simulink model "BaseEngineController_LS_128"  (Simulink 7.7)
settings: Solver=FixedStepDiscrete  StartTime=0.0  StopTime=10.0  RelTol=1e-3
PreLoadFcn:
  | try, eval([bdroot '_setup']); catch, eval('model_setup', ''); end
InitFcn:
  | try, eval([bdroot '_setup']); catch, eval('model_setup', ''); end
undefined symbols (not defined in the file): ECU565, High, motohawk_build_version, motohawk_trunc_name, motohawk_vardec_config_group, motohawk_vardec_path, True
libraries: MotoHawk_lib x1418, motohawk_control_primitives_lib x183, motohawk_engine_lib x32, simulink x21, motohawk_annotations_lib x9, AutoDoc_lib x8, simulink_extras x4, motohawk_ccp_examples_lib x1, motohawk_control_primitives_motoshare_lib x1
(part 1 of 27)
Description:
  | MI07 SECM48
CloseFcn:
  | rtwprivate ssgencode ModelCloseRequest BaseEngineController_A02
settings Model: MotoHawkBuildVersion=035  MotoHawkBuildStats=struct('TotalFLASH',{373552},'TotalEEPROM',{1254},'TotalRAM',{26040},'AppFLASH',{154160},'AppEEPROM',{1080},'AppRAM',{7766},'HeapRAM',{4096},'BuildSuccessCount',{48},'BuildErrorCount',{105},'OSRAM',{4962},'StackRAM',{9216},'FgndTimeStackSize',{4096},'FgndAngleStackSize',{1024},'BgndStackSize',{2048},'IdleStackSize',{1024},'InterruptStackSize',{1024},'RTWBlockIOSize',{2192},'RTWDWorkSize',{1776},'RTWPrevZCSize',{0},'VolatileSize',{1668},'NonVolatileSize',{1080},'ConstantSize',{18616},'NonVolatileFormatID',{32179})  MotoHawkModelSavedName=BaseEngineController_LS_128  MotoHawkModelGUID=a749ec14-8a37-4ecf-bb-ef-07-f5-29-2a-95  MotoHawkModelOpenTime=2022 11 22 13 19 39.99  MotoHawkModelElapsedTime=-3851959716.408  MotoHawkBuildGUID=70e4bce9-a719-451e-bc-76-a9-56-b2-7d-46  MotoHawkBuildInfo=struct('model_name',{'BaseEngineController_LS_128'},'motohawk_version',{'2011a_sp0.184'},'motohawk_component_version',{'0.0.7'},'matlab_version',{'7.12.0'},'build_version',{'034'},'module_type',{'ECU565-128'},'layout_type',{'DEV'},'processor_family',{'PPC'},'processor_type',{'MPC565'},'toolchain_vendor',{'gcc-powerpc-eabi'},'toolchain_version',{'4.4.0'},'component',{0},'archive_file',{'PCM128.a'},'enable_build',{1},'fptype',{0},'flash_size',{1048576},'ee_size',{8192},'ram_size',{36864},'decram_size',{4096},'module_memory_def',{'MPC565_ModMemoryDef_Dev'},'eri_table0_rev',{9},'max_eri_table_size',{65535},'use_debug_vardecs',{1},'use_info_vardecs',{1},'fgnd_base_period_ms',{5},'bgnd_base_period_ms',{50},'root_build_dir',{'C:\Users\maxar\Documents\GitHub\Engine-Controller\EngineController_128Branch'},'build_dir',{'C:\Users\maxar\Documents\GitHub\Engine-Controller\EngineController_128Branch\BaseEngineController_LS_128_Build'},'dll_name',{'BaseEngin_034'},'srz_name',{'BaseEngineController_LS_128_034'},'fgnd_stack_size',{4096},'fgnd_angle_stack_size',{0},'bgnd_stack_size',{1024},'idle_stack_size',{1024},'irq_stack_size',{1280},'heap_size',{2048},'heap_margin',{409},'install_dll_dir',{'c:\ecufiles\tdbdll'},'install_srz_dir',{'C:\ECUFiles\Programs\'},'app_int_stack_size',{1024},'shutdown_stack_size',{1024},'mingw_dir',{'C:\PROGRA~2\Woodward\DEVELO~1\TOOLCH~1\GCC\win32-pe\4_4_0\'},'motohawk_dir',{'C:\PROGRA~2\Woodward\MCS\MotoHawk\2011A_~1.184'},'toolchain_dir',{'C:\Program Files (x86)\Woodward\DevelopmentTools\Toolchains\GCC\powerpc-eabi\4_4_0\'},'matlab_root',{'E:\MATLAB\2011a'},'model_guid',{'a749ec14-8a37-4ecf-bb-ef-07-f5-29-2a-95'},'build_guid',{'70e4bce9-a719-451e-bc-76-a9-56-b2-7d-46'},'token_guid',{'DD8AD11F95A6FC42BFF9AC780840E4B4'})  RegisteredStructs=struct('Name',{'FreezeFrame','FreezeFrames'},'Data',{struct('Name',{int32(0)},'Code',{int32(0)},'Var1',{int32(0)},'Var2',{int32(0)},'Var3',{int32(0)},'Var4',{int32(0)},'Var5',{int32(0)},'Var6',{int32(0)},'Var7',{int32(0)},'Var8',{int32(0)},'Var9',{int32(0)},'Var10',{int32(0)}),struct('Name',{int32(0)},'Code',{int32(0)},'Var1',{int32(0)},'Var2',{int32(0)},'Var3',{int32(0)},'Var4',{int32(0)},'Var5',{int32(0)},'Var6',{int32(0)},'Var7',{int32(0)},'Var8',{int32(0)},'Var9',{int32(0)},'Var10',{int32(0)})},'Enums',{{{'None','APP_Sensors_Conflict','CamEdgesFault','CamSyncFault','CrankEdgesFault','CrankSyncFault','ECTOverTempFault','ECTRangeHigh','ECTRangeLow','ECT_IR_Fault','EST1_Open','EST1_Short','EST2_Open','EST2_Short','EST3_Open','EST3_Short','EST4_Open','EST4_Short','EST5_Open','EST5_Short','EST6_Open','EST6_Short','EST7_Open','EST7_Short','EST8_Open','EST8_Short','ETCSpringTest','ETC_Open_Fault','ETC_Sticking','FuelAdaptRangeHi','FuelAdaptRangeLow','FuelTempRangeHigh','FuelTempRangeLow','HBridgeFault_ETC','HardOverspeed','IATRangeHigh','IATRangeLow','IAT_IR_Fault','Inj1Open','Inj2Open','Inj3Open','Inj4Open','Inj5Open','Inj6Open','Inj7Open','Inj8Open','LSDFault_FuelPump','LSDFault_MIL','LSOFault_VVT','MAFRangeHigh','MAFRangeLow','MAPRangeHigh','MAPRangeLow','MAPTimeRangeHigh','MAPTimeRangeLow','MAP_IR_HI','MAP_IR_LO','MAP_STICKING','MediumOverspeed','O2FailedLean','O2FailedRich','O2NotActive','OilTempRangeHigh','OilTempRangeLow','SensVoltRangeHigh','SensVoltRangeLow','SoftOverspeed','SysVoltRangeHigh','SysVoltRangeLow','TPS_Sensors_Conflict'}},{{'None','CamEdgesFault','CamSyncFault','CrankEdgesFault','CrankSyncFault','ECTOverTempFault','ECTRangeHigh','ECTRangeLow','ECTSevereOverTempFault','EGRSenseRangeHigh','EGRSenseRangeLow','EST1_Open','EST1_Short','EST2_Open','EST2_Short','ETCSpringTest','ETC_Open_Fault','ETC_Sticking','FuelAdaptRangeHi','FuelAdaptRangeLow','FuelPresHigh_Fault','FuelPresLow_Fault','FuelPresRangeHigh','FuelPresRangeLow','FuelSensRangeHigh','FuelSensRangeLow','HBridgeFault_ETC','HardOverspeed','IATRangeHigh','IATRangeLow','Inj1Open','Inj2Open','LSDFault_FuelPump','LSDFault_OilPump','LSDFault_OxygenHeater','MAFRangeHigh','MAFRangeLow','MAPRangeHigh','MAPRangeLow','MAPTimeRangeHigh','MAPTimeRangeLow','MAP_IR_HI','MAP_IR_LO','MAP_STICKING','MediumOverspeed','NoOil_Fault','O2FailedLean','O2FailedRich','O2NotActive','O2_PostCatRangeHigh','O2_PostCatRangeLow','OilPresRangeHigh','OilPresRangeLow','SensVoltRangeHigh','SensVoltRangeLow','SoftOverspeed','SysVoltLow_Fault','SysVoltRangeHigh','SysVoltRangeLow','TPS1AdaptHiMax','TPS1AdaptHiMin','TPS1AdaptLoMax','TPS1AdaptLoMin','TPS1RangeHigh','TPS1RangeLow','TPS2AdaptHiMax','TPS2AdaptHiMin','TPS2AdaptLoMax','TPS2AdaptLoMin','TPS2RangeHigh','TPS2RangeLow','TPS_Sensors_Conflict'}}})  Creator=dbocci  LastModifiedBy=maxar
settings OptimizationCC: InlineParams=on  InitFltsAndDblsToZero=on  OptimizeModelRefInitCode=on  LifeSpan=1
settings DebuggingCC: SolverPrmCheckMsg=none  InheritedTsInSrcMsg=none  TasksWithSamePriorityMsg=none  StrictBusMsg=Warning
settings HardwareCC: ProdEndianess=BigEndian  ProdHWDeviceType=Specified
settings RTWCC: SystemTargetFile=motohawk_ert_rtw.tlc  TLCOptions="-aCustomNonFinites=\"motohawk_genrtnonfinite.tlc\""  MakeCommand=motohawk_make_rtw  TemplateMakefile=motohawk_ert_rtw.tmf  Description=MotoHawk(tm) Rapid Prototyping  ProcessScript=motohawk_ert_rtw_make_rtw_hook
settings CodeAppCC: IgnoreCustomStorageClasses=off  MaxIdLength=100  CustomSymbolStrField=$H$N$M
settings STFCustomTargetCC: FunctionExecutionProfile=off  ModelReferenceCompliant=off  CombineOutputUpdateFcns=on  ERTCustomFileBanners=on  SupportContinuousTime=off  SupportNonInlinedSFcns=off  SystemTargetFile=motohawk_ert_rtw.tlc
settings ERTTargetCC: FunctionExecutionProfile=off  MultiwordLength=2048  ModelReferenceCompliant=off  ParMdlRefBuildCompliant=off  CompOptLevelCompliant=off  ERTFirstTimeCompliant=off  ModelStepFunctionPrototypeControlCompliant=off  CPPClassGenCompliant=off  ERTCustomFileTemplate=example_file_process.tlc  ConvertIfToSwitch=off

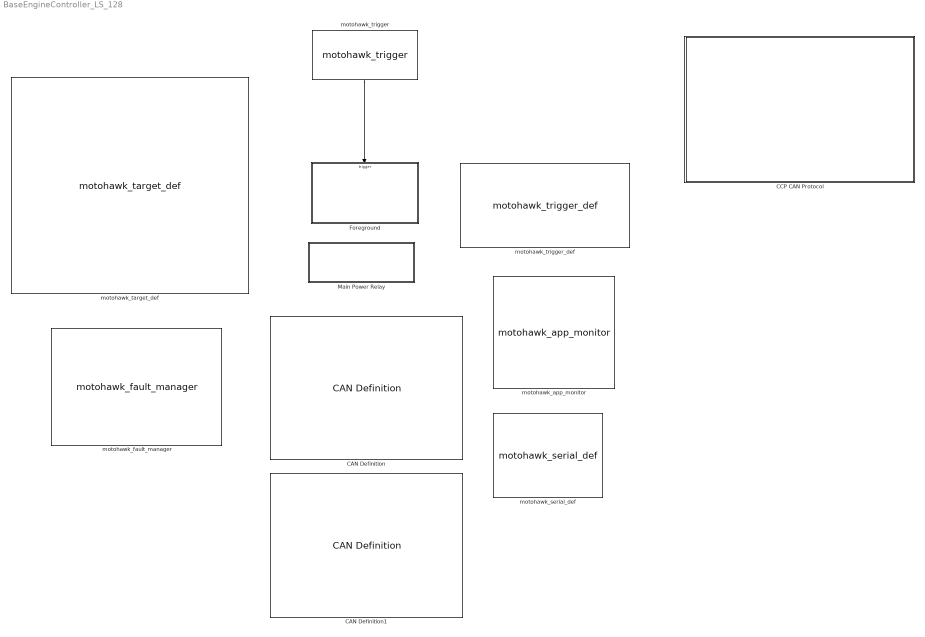
== system BaseEngineController_LS_128 ==
  CAN Definition : MotoHawk_lib/CAN Blocks/CAN Definition  Priority=-100  nam=['CAN_1']  text_resource=CAN1  code_resource=NONE  val_resource=-1  target=ECU565-128  bus=-2  btime=500 kbaud  pre=1  prop=0  pseg1=0  pseg2=0  resyn=0  tx_queue_size=16  rx_queue_size=16  use_protocol=on  city_id=hex2dec('B')  access_level=4  mototune_group='System | System Config | Communication Config'
  CAN Definition1 : MotoHawk_lib/CAN Blocks/CAN Definition  Priority=-100  nam=['CAN_2']  text_resource=CAN2  code_resource=NONE  val_resource=-1  target=ECU565-128  bus=-2  btime=500 kbaud  pre=1  prop=0  pseg1=0  pseg2=0  resyn=0  tx_queue_size=16  rx_queue_size=16  use_protocol=on  city_id=hex2dec('B')  access_level=4  mototune_group='System | System Config | Communication Config'
  CCP CAN Protocol : Subsystem  AncestorBlock=MotoHawk_lib/CCP Slave/CCP CAN Protocol  mask(MotoHawk CCP CAN Protocol Handler){image_file='ccp.jpg', mtninstance='CCP1', stataddr=hex2dec('31'), channel_name='CAN_1', channel=-2, rxid=hex2dec('18ef0231'), rxidtype=1, rxidmasknom=hex2dec('1fffffff'), txid=hex2dec('18ef3102'), txidtype=1, daqs=10, odts=8, nvodt=2, send_cpb_resp=on, use_mototune_group=on, mototune_group=['System | CCP | ', motohawk_get_param_ws(gcb, 'mtninstance')]}
      mask prompts: image_file "imfileImage File"; mtninstance "CCP Handler Instance Name (unique string)"; stataddr "CCP Station Address (16 bit integer)"; channel_name "CAN Channel Name"; channel "CAN Channel (integer)"; rxid "Receive ID (CRO)"; rxidtype "Receive ID Type (0=Std, 1=Ext)"; rxidmasknom "Receive ID Mask"; txid "Transmit ID (DTO/DAQ)"; txidtype "Transmit ID Type (0=Std, 1=Ext)"; daqs "Total Number of DAQs [1-253]"; odts "Total Number of Object Descriptors (ODT ) per DAQ [1-253]"; nvodt "Store ODTs in Non Volatile (0=RAM, 1=EEPROM, 2=CAL)"; send_cpb_resp "Send "Command Processor Busy" response prior to long memory writes"; use_mototune_group "------ Show MotoTune Group ------"; mototune_group "MotoTune Group String"
      mask help:
      | Handle a CCP connection via CAN.
      |
      | The list of DAQ Triggers is pre-selected to:
      |  o FGND_RTI_PERIODIC
      |  o FGND_2XRTI_PERIODIC
      |  o FGND_10XRTI_PERIODIC
      |  o FGND_20XRTI_PERIODIC
      |  o BGND_BASE_PERIODIC
      |  o BGND_BASEx2_PERIODIC
      |  o BGND_BASEx10_PERIODIC
      |  o ONE_SECOND_EVENT
      |
      | The CCP Command packets are responded to in the CAN interrupt in which they occur.
      | If you would like other triggering behavior, please utilize the CCP CAN Protocol External Trig
      | block from the CCP Slave Library.
      |
      | Support operations:
      | Upload Calibrations
      | Download Calibrations
      | Data Acquisition
      | Seed and Key security
      |
      | Not Supported:
      | Flashing operations
      |
      | --------------------------------------------------------------------------------
      | Copyright 2010 Woodward.  All Rights Reserved.
      mask init:
      | block = gcb;
      | try,
      | 	img = imread(image_file);
      | 	%motohawk_block_image(gcb, image_file);
      | catch,
      | 	img = imread('image_not_found.jpg');
      | end
      | 
      | if channel > -1
      | 	%% Automatically upgrade the nam parameter if the bus is currently set to a channel number
      | 	bus_expr = get_param(block, 'channel');
      | 	% Note, the set_param within the upgrade function will fail, we do the set_param next
      | 	[nam,expr] = motohawk_upgrade_can_name('', channel, bus_expr);
      | 
      | 	try
      | 		set_param(block, 'channel_name', expr, 'channel', '-2');
      | 	end
      | end
      | 
      | e = {'(std)','(ext)'};
      | o = {'RAM','EEPROM','CAL'};
      | 
      | if((nvodt > 2) || (nvodt < 0))
      | 	set_param(gcb,'nvodt','0');	
      | end
      | 
      | nvlbl = ['ODT Storage: ' o{nvodt+1}];
      | 
      | reqbits = hex2dec('1fffffff'); 
      | rxidmask = bitand(uint32(rxidmasknom),uint32(reqbits));
      | rxlbl = sprintf('\\fontname{courier new}Chan  : %s\\newlineRx ID : 0x%08x %s\\newlineID Adj: 0x%08x', motohawk_tex(channel_name),rxid,e{rxidtype+1}, double(bitxor(uint32(rxidmask),uint32(reqbits))));
      | txlbl = sprintf('\\fontname{courier new}Chan  : %s\\newlineTx ID : 0x%08x %s\\newline ', motohawk_tex(channel_name),txid,e{txidtype+1});
      settings: MoveFcn=%motohawk_block_image(gcb, motohawk_get_param_ws(gcb, 'image_file'));
      mask Help: eval('motohawk_block_help(get_param(gcb,''MaskType''))');
      mask CallbackString: |||||||||||||motohawk_set_param([gcb '/CCP CAN Protocol External Trig1'], 'send_cpb_resp', get_param(gcb, 'send_cpb_resp'));|motohawk_calibration_visible(gcb, 'use_mototune_group');|
      mask Display:
      | patch([0 0 1 1], [0 1 1 0], [220/255 220/255 220/255]);
      | patch([0 0 1 1], [0 0.075 0.075 0], [230/255 0/255 0/255]);
      | patch([0 0 1 1], [0.025 0.05 0.05 0.025], [150/255 0/255 0/255]);
      | patch([0 0 1 1], [0 0.025 0.025 0], [0/255 0/255 0/255]);
      | image(img,[0.05 0.3 0.55 0.7]);
      | 
      | text(0.99,0.57,['\fontname{Arial}\fontsize{18}\bfCCP Handler\fontsize{12}\newline\rmInstance: ' strrep(mtninstance,'_','\_') '\newlineStation Addr: ' sprintf('0x%04x',stataddr) '\newlineDAQs: ' sprintf('%g',daqs) '\newlineODTs: ' sprintf('%g',odts) '\newline' nvlbl],'texmode','on','HorizontalAlignment','Right');
      | 
      | text(0.01,0.22,['\fontname{Arial}\fontsize{18}\bfRx\fontsize{12}\newline\rm' rxlbl],'texmode','on','HorizontalAlignment','Left');
      | text(0.99,0.22,['\fontname{Arial}\fontsize{18}\bfTx\fontsize{12}\newline\rm' txlbl],'texmode','on','HorizontalAlignment','Right');
  Foreground : Subsystem  TreatAsAtomicUnit=on
      settings: RTWSystemCode=Function  RTWFcnNameOpts=Use subsystem name  RTWFileNameOpts=Use subsystem name
  Main Power Relay : Subsystem  AncestorBlock=MotoHawk_lib/Extra Development Blocks/Main Power Relay  mask(MotoHawk Main Power Relay Control){on_delay_count=2, off_delay_count=5, group='System | Main Power Relay'}
      mask prompts: on_delay_count "On Delay Count"; off_delay_count "Off Delay Count"; group "MotoTune Group"
      mask help:
      | This block provides basic control of the main power relay, by following the ECUP voltage input pin.
      |
      | Regardless of where the block is placed in a design, the strategy will execute every 50ms with background priority.
      |
      | Note that this block is simply composed of other primitive MotoHawk blocks and may be used as a starting point for a more complicated strategy.
      |
      | On Delay:  Once the ECU power goes high, after this period, the Main Power Relay will be turned on.
      | Off Delay:  Once the ECU power goes low, after this period, the Main Power Relay will be turned off.
      |
      | Note that one tick before MPRD is turned off, non-volatile variables will be stored, and the Shutdown event will be posted.  It is not necessary to use the Shutdown event.
      |
      | To delay shutdown based on Foreground events, use a data storage write block 'ShutDownTasksComplete' set as a boolean in the Foreground controller to initiate actual shutdown following completion of the tasks.
      |
      | ---------------------------------------------------------------------
      | Copyright 2005 MotoTron, Inc.  All Rights Reserved.
      mask init:
      | on_delay_lbl = sprintf('\nOn Delay: %d ms', on_delay_count * 50);
      | off_delay_lbl = sprintf('\nOff Delay: %d ms', off_delay_count * 50);
      mask Help: eval('motohawk_block_help(get_param(gcb,''MaskType''))');
      mask Display:
      | patch([0 0 1 1], [0 1 1 0], [220/255 220/255 220/255])
      | patch([0 0 1 1], [0 0.075 0.075 0], [230/255 0/255 0/255])
      | patch([0 0 1 1], [0.025 0.05 0.05 0.025], [150/255 0/255 0/255])
      | patch([0 0 1 1], [0 0.025 0.025 0], [0/255 0/255 0/255])
      | 
      | disp(['Main Power Relay' on_delay_lbl off_delay_lbl]);
  motohawk_app_monitor : MotoHawk_lib/System Debug Blocks/motohawk_app_monitor  fgnd_stack_margin=512  fgnd_angle_stack_margin=256  bgnd_stack_margin=256  idle_stack_margin=256  irq_stack_margin=128  heap_margin=256  cpu_margin=10  init_enable=Enabled  pause_point=Do Not Pause on Startup
  motohawk_fault_manager : MotoHawk_lib/Fault Management Blocks/motohawk_fault_manager  storage=FLASH  read_level=1  write_level=1  clear_level=1  xytype=uint16  mototune_group=motohawk_vardec_path(gcb)
  motohawk_serial_def : MotoHawk_lib/Serial I//O Blocks/motohawk_serial_def  res_name=[]  text_resource=RS485  code_resource=NONE  val_resource=-1  target=ECU565-128  resource_enum_str=(None)=-1,RS485=113  use_mototune=on  baud=9600  tx_queue_size=16  rx_queue_size=16
  motohawk_target_def : MotoHawk_lib/motohawk_target_def  Priority=-65535  target=ECU565-128  layout=DEV  fptype=single (32 bits)  fgnd_stack_size=4*1024  fgnd_angle_stack_size=0  bgnd_stack_size=1*1024  idle_stack_size=1024  irq_stack_size=1280  app_int_stack_size=1024  shutdown_stack_size=1024  heap_size=2*1024  show_margins=off  fgnd_stack_margin=(3*1024) * 0.1  fgnd_angle_stack_margin=0  bgnd_stack_margin=(2*1024) * 0.1  idle_stack_margin=(1024) * 0.1  irq_stack_margin=(1536) * 0.1  app_int_stack_margin=(1024) * 0.1  shutdown_stack_margin=(1024) * 0.1  heap_margin=(4*1024) * 0.1  comp_name=bdroot  comp_img='mh.jpg'  comp_security=No Encryption  comp_build_pass='mhbuild'  comp_sim_pass='mhsim'  comp_multi=off  show_filenames=on  dll_name=motohawk_trunc_name(bdroot, ['_' motohawk_build_version], 13)  srz_name=motohawk_trunc_name(bdroot, ['_' motohawk_build_version], 50)  build_dir=''  comp_dir='.'
  motohawk_trigger : MotoHawk_lib/Trigger Blocks/motohawk_trigger  Tag=Trigger  Priority=0  trigger=FGND_RTI_PERIODIC  function_name=Trigger_FGND_RTI_PERIODIC_11578p0004  priority_order=0  inherited=off  run_disabled=off  override_app_monitor=off  target=ECU565_128
  motohawk_trigger_def : MotoHawk_lib/Trigger Blocks/motohawk_trigger_def  fgnd_rti_rate=5000  bgnd_base_multiple=10  read_level=1  write_level=1  mototune_group='System | System Config | Trigger Config'
  wires:
  motohawk_trigger/1 -> Foreground/Trigger

== system BaseEngineController_LS_128/CCP CAN Protocol ==
  CCP CAN Protocol External Trig1 : MotoHawk_lib/CCP Slave/CCP CAN Protocol External Trig  SystemSampleTime=-1  image_file=image_file  mtninstance=mtninstance  stataddr=stataddr  channel_name=channel_name  channel=channel  rxid=rxid  rxidtype=rxidtype  rxidmasknom=rxidmasknom  txid=txid  txidtype=txidtype  daqs=daqs  odts=odts  nvodt=nvodt  send_cpb_resp=on  use_mototune_group=off  mototune_group=mototune_group
  CCP Triggers : motohawk_ccp_examples_lib/CCP Triggers  SystemSampleTime=-1
      link override motohawk_trigger: trigger=FGND_5XRTI_PERIODIC  function_name=Trigger_FGND_5XRTI_PERIODIC_23675p0006  target=ECU555_80
      link override motohawk_trigger2: trigger=FGND_MID_TDC_EVENT  function_name=Trigger_FGND_MID_TDC_EVENT_23677p0006  target=ECU555_80
  motohawk_trigger1 : MotoHawk_lib/Trigger Blocks/motohawk_trigger  Tag=Trigger  trigger=IDLE_EVENT  function_name=Trigger_IDLE_EVENT_9p001  priority_order=255  inherited=on  run_disabled=off  override_app_monitor=on  target=ECU565_128
  wires:
  motohawk_trigger1/1 -> CCP CAN Protocol External Trig1/1
  CCP Triggers/1 -> CCP CAN Protocol External Trig1/2

== system BaseEngineController_LS_128/Foreground ==
  f : TriggerPort  TriggerType=function-call
  Control : Subsystem  mask(Display Image File){image_file='pcm555.jpg'}
      mask prompts: image_file "Image File"
      mask help:
      | Enter an image file on the current MATLAB path to display on this block.
      |
      | Double-clicking this block opens the contents of the subsystem.  Right-click and select 'Mask parameters...' to select a new image file.
      |
      | To use just the mask of this block in a model, but supply your own contents, break the link to the library.
      mask init:
      | try,
      | 	img = imread(image_file);
      | 	motohawk_block_image(gcb, image_file);
      | catch,
      | 	img = imread('image_not_found.jpg');
      | end
      settings: OpenFcn=open_system(gcb,'force')  MoveFcn=motohawk_block_image(gcb, motohawk_get_param_ws(gcb, 'image_file'));
      mask Display: image(img);
  Inputs : Subsystem  mask(Display Image File){image_file='sensor.jpg'}
      mask prompts: image_file "Image File"
      mask help:
      | Enter an image file on the current MATLAB path to display on this block.
      |
      | Double-clicking this block opens the contents of the subsystem.  Right-click and select 'Mask parameters...' to select a new image file.
      |
      | To use just the mask of this block in a model, but supply your own contents, break the link to the library.
      mask init:
      | try,
      | 	img = imread(image_file);
      | 	motohawk_block_image(gcb, image_file);
      | catch,
      | 	img = imread('image_not_found.jpg');
      | end
      settings: OpenFcn=open_system(gcb,'force')  MoveFcn=motohawk_block_image(gcb, motohawk_get_param_ws(gcb, 'image_file'));
      mask Display: image(img);
  Outputs : Subsystem  mask(Display Image File){image_file='actuator.jpg'}
      mask prompts: image_file "Image File"
      mask help:
      | Enter an image file on the current MATLAB path to display on this block.
      |
      | Double-clicking this block opens the contents of the subsystem.  Right-click and select 'Mask parameters...' to select a new image file.
      |
      | To use just the mask of this block in a model, but supply your own contents, break the link to the library.
      mask init:
      | try,
      | 	img = imread(image_file);
      | 	motohawk_block_image(gcb, image_file);
      | catch,
      | 	img = imread('image_not_found.jpg');
      | end
      settings: OpenFcn=open_system(gcb,'force')  MoveFcn=motohawk_block_image(gcb, motohawk_get_param_ws(gcb, 'image_file'));
      mask Display: image(img);
  wires:
  Control/1(Actuators) -> Outputs/1(Actuators)
  Inputs/1(SensorBus) -> Control/1(Sensors)

== system BaseEngineController_LS_128/Main Power Relay ==
  note: The saving and restoring of non-volatile variables
      | must be called from a background priority task.
  note: Always execute Main Power Relay control in the background.
  Main Power Relay : Subsystem  TreatAsAtomicUnit=on
  motohawk_trigger : MotoHawk_lib/Trigger Blocks/motohawk_trigger  Tag=Trigger  Priority=255  trigger=BGND_BASE_PERIODIC  function_name=Trigger_BGND_BASE_PERIODIC_11570p0004  priority_order=255  inherited=on  run_disabled=on  override_app_monitor=off  target=ECU565_128
  wires:
  motohawk_trigger/1 -> Main Power Relay/Trigger

== system BaseEngineController_LS_128/Foreground/Control ==
  Sensors : Inport
  ActuatorCharacterization : Subsystem
  Controller : Subsystem
  Diagnostics : Subsystem  TreatAsAtomicUnit=on
  VirtualSensors : Subsystem
      settings: RTWSystemCode=Function  RTWFcnNameOpts=Use subsystem name  RTWFileNameOpts=Use function name
  motohawk_function_collector : MotoHawk_lib/Extra Development Blocks/motohawk_function_collector  SystemSampleTime=-1  count=5
  Actuators : Outport
  wires:
  Sensors/1 -> VirtualSensors/1(Raw)
  VirtualSensors/1(Sensors) -> Controller/1(Sensors), ActuatorCharacterization/2(Sensors), Diagnostics/2(Sensors)
  ActuatorCharacterization/1(Actuators) -> Actuators/1
  Controller/1(Actuators) -> ActuatorCharacterization/1(Control), Diagnostics/1(Control)
  Diagnostics/1(Diagnostics) -> ActuatorCharacterization/3(Diagnsotics)
  motohawk_function_collector/1 -> Diagnostics/Trigger
  Controller/2(DesEquivRatio) -> Diagnostics/3(DesEquivRatio)

== system BaseEngineController_LS_128/Foreground/Inputs ==
  Bus Creator : BusCreator  Inputs=7
  CAN : Subsystem
  Digital : Subsystem
  EngineSpeed : Subsystem
  LinearSensors : Subsystem
  NonLinearSensors : Subsystem
  PotentiometerSensors : Subsystem
  SensorBus : Outport
  wires:
  Digital/1(SensorBus) -> Bus Creator/6
  PotentiometerSensors/1(SensorBus) -> Bus Creator/5
  NonLinearSensors/1(SensorBus) -> Bus Creator/4
  LinearSensors/1(SensorBus) -> Bus Creator/3
  EngineSpeed/2(RPM) -> Bus Creator/2  "RPM"
  EngineSpeed/1(RPMInst) -> Bus Creator/1  "RPMInst"
  Bus Creator/1 -> SensorBus/1
  CAN/1(SensorBus) -> Bus Creator/7  "CAN"

== system BaseEngineController_LS_128/Foreground/Outputs ==
  Actuators : Inport
  AC Control : Subsystem
  AEM Infinity Dash : Subsystem
  Bus Selector : BusSelector  OutputSignals=Controller.WASTEGATE
  Bus Selector1 : BusSelector  OutputSignals=Controller.FUELP,Sensors.Raw.Digital.ESTOP
  Bus Selector2 : BusSelector  OutputSignals=Controller.IAC-P,Controller.IAC-S
  Bus Selector3 : BusSelector  OutputSignals=ActuatorCharacterization.ETC,Sensors.RawIndexes.SysVolt09Idx,Sensors.Raw.Digital.ESTOP,Sensors.RawProcessed.TimeSinceStall
  Bus Selector4 : BusSelector  OutputSignals=Controller.SOI,ActuatorCharacterization.InjMPW,ActuatorCharacterization.InjEPWOffset,ActuatorCharacterization.FuelCutSeq,Controller.MakeUpEOI
  Bus Selector5 : BusSelector  OutputSignals=ActuatorCharacterization.SparkEnable,ActuatorCharacterization.SparkStartAngle,Controller.SparkAdv,ActuatorCharacterization.SparkCutSeq
  Bus Selector6 : BusSelector  OutputSignals=Controller.FAN-1,Controller.FAN-2
  Bus Selector7 : BusSelector  OutputSignals=Controller.AC
  Coil Control : Subsystem  TreatAsAtomicUnit=on
  Documentation_Calibrations_Probes_Block : AutoDoc_lib/Documentation_Calibrations_Probes_Block
  Documentation_Left_Border : AutoDoc_lib/Documentation_Left_Border  layout=Portrait
  ETC_CutPower : Subsystem
  FAN Control : Subsystem
  FuelPump : Subsystem
  HBridge : Subsystem
  IAC-Control : Subsystem
  Injector Control : Subsystem
  Logical Operator4 : Logic  Operator=NOT  AllPortsSameDT=off  OutDataTypeStr=boolean
  Logical Operator5 : Logic  AllPortsSameDT=off  OutDataTypeStr=boolean
  WASTEGATE-Control : Subsystem
  motohawk_trigger : MotoHawk_lib/Trigger Blocks/motohawk_trigger  Tag=Trigger  trigger=FGND_5XRTI_PERIODIC  function_name=Trigger_FGND_5XRTI_PERIODIC_11294p0006  priority_order=1  inherited=on  run_disabled=off  override_app_monitor=off  target=ECU565_128
  wires:
  Bus Selector3/2 -> HBridge/2(SysVoltIdx)  "<SysVolt09Idx>"
  Bus Selector4/5 -> Injector Control/5(MakeUpEOI)  "<MakeUpEOI>"
  Bus Selector3/1 -> HBridge/1(ETCDuty Cycle), ETC_CutPower/1(ETC)  "<ETC>"
  Bus Selector5/4 -> Coil Control/4(CutSequence)  "<SparkCutSeq>"
  Bus Selector4/4 -> Injector Control/4(CutSequence)  "<FuelCutSeq>"
  Bus Selector5/3 -> Coil Control/3(SparkAdvance)  "<SparkAdv>"
  Bus Selector5/2 -> Coil Control/2(SparkStartAngle)  "<SparkStartAngle>"
  Bus Selector4/3 -> Injector Control/3(InjEPWOffset)  "<InjEPWOffset>"
  Bus Selector4/2 -> Injector Control/2(InjMPW)  "<InjMPW>"
  Bus Selector5/1 -> Coil Control/1(SparkEnable)  "<SparkEnable>"
  Bus Selector4/1 -> Injector Control/1(SOI)  "<SOI>"
  Actuators/1 -> Bus Selector3/1, Bus Selector1/1, Bus Selector2/1, Bus Selector/1, Bus Selector6/1, Bus Selector7/1, AEM Infinity Dash/1(Data), Bus Selector5/1, Bus Selector4/1
  motohawk_trigger/1 -> Coil Control/Trigger
  Bus Selector1/2 -> Logical Operator4/1  "<ESTOP>"
  Logical Operator4/1 -> Logical Operator5/2
  Bus Selector1/1 -> Logical Operator5/1  "<FUELP>"
  Logical Operator5/1 -> FuelPump/1(State)
  Bus Selector2/1 -> IAC-Control/1(IAC-P)  "<IAC-P>"
  Bus Selector2/2 -> IAC-Control/2(IAC-S)  "<IAC-S>"
  Bus Selector/1 -> WASTEGATE-Control/1(WASTEGATE)  "<WASTEGATE>"
  Bus Selector6/1 -> FAN Control/1(FAN-1)  "<FAN-1>"
  Bus Selector6/2 -> FAN Control/2(FAN-2)  "<FAN-2>"
  Bus Selector7/1 -> AC Control/1(AC)  "<AC>"
  ETC_CutPower/1(ETC OFF) -> HBridge/3(ETC_CutPower)
  Bus Selector3/3 -> ETC_CutPower/2(ESTOP)  "<ESTOP>"
  Bus Selector3/4 -> ETC_CutPower/3(TimeSinceStall)  "<TimeSinceStall>"

== system BaseEngineController_LS_128/Main Power Relay/Main Power Relay ==
  note: Provide Data Store
      | Access to MPRD State
  note: Control Main Power Relay
  note: NonVolatile Memory Store/Restore
      | Hooks from MotoTune
  note: Software Reset
      | Hook from MotoTune
  note: When ProcessorReboot goes true, it will force a falling edge to perform a shutdown, save NV vars, shutdown power, and then cause a processor reset if still true
  note: After a delay, turn on or off Main Power Relay
  f : TriggerPort  TriggerType=function-call  SampleTime=-1  ZeroCross=off
  Display Variable Event Boolean : MotoHawk_lib/Extra Development Blocks/Display Variable Event Boolean  SystemSampleTime=-1  nam='ProcessorReboot'  level=1  enum_str={'Run', 'Reboot'}  help_str='Reboots the processor when set.'  group=group
  Display Variable Event Function-Call : MotoHawk_lib/Extra Development Blocks/Display Variable Event Function-Call  SystemSampleTime=-1  nam='RestoreNVFactoryDefaults'  level=1  enum_str={'Run', 'Restore To Defaults'}  help_str='Restores NonVolatile Memory to Factory Defaults'  group='System | NonVolatile Storage'
  Display Variable Event Function-Call1 : MotoHawk_lib/Extra Development Blocks/Display Variable Event Function-Call  SystemSampleTime=-1  nam='StoreNV'  level=1  enum_str={'Run', 'Store To EEPROM'}  help_str='Stores RAM-Shadowed memory to serial EEPROM'  group='System | NonVolatile Storage'
  ECUP Latch : Stateflow chart  TreatAsAtomicUnit=on
  Forced Shutdown Process : Subsystem
  Logical Operator : Logic
  Logical Operator1 : Logic  Operator=NOT
  Logical Operator2 : Logic  Inputs=3
  Logical Operator3 : Logic  Operator=NOT  AllPortsSameDT=off  OutDataTypeStr=boolean
  On Off Delay : Subsystem
  Relational Operator : RelationalOperator  ZeroCross=off  InputSameDT=on
  Relational Operator1 : RelationalOperator  ZeroCross=off  InputSameDT=on
  ShutDown Processes : Subsystem
  Time Since Enabled (With Input)1 : motohawk_control_primitives_lib/Time Since Enabled (With Input)1  SystemSampleTime=-1  nam='TimeSinceShutdown'  samp_time=-1  init=0  upperlim=16000
  Unit Delay3 : UnitDelay  SampleTime=-1
  Unit Delay4 : UnitDelay  SampleTime=-1
  Unit Delay5 : UnitDelay  SampleTime=-1
  motohawk_ain5 : MotoHawk_lib/Analog I//O Blocks/motohawk_ain  res_name=[]  text_resource=ECUP  code_resource=RES_ECUP  val_resource=-1  target=ECU565-128  resource_enum_str=(None)=-1,ECUP=53,DRVP=54,XDRP=55,AN1M=56,AN2M=57,AN3M=58,AN4M=59,AN5M=60,AN6M=61,AN7M=62,AN8M=63,AN9M=64,AN10M=65,AN11M=66,AN12M=67,AN13M=68,AN14M=69,AN15M=70,AN16M=71,AN17M=72,AN18M=73,AN19M=74,AN20M=75,AN21M=76,AN22M=77,AN23M=78,AN24M=79,AN25M=80,AN26M=81,AN27M=82,AN28M=83,AN29M=84,AN30M=85,AN31M=86,AN32M=87,AN33M=88,AN34M=89,O2A=90,O2B=91,XDRP_B=92,REF_14V=143  altref=5V Reference  typ=uint16  num_adc_bits=10  use_stat=off  use_vardec=off  nam='AIN'  read_level=1  write_level=1  group='System | I/O Pins | Inputs Config'
  motohawk_calibration : MotoHawk_lib/Calibration & Probing Blocks/motohawk_calibration  nam='ECUP_Threshold'  val=100  storage=Calibration  show_more=on  name_source=Use Parameter  data_type=Inherit via back propagation  read_level=1  write_level=1  ovr_cals=on  view_as=Number  enum_struct={'Disabled', 'Enabled'}  vector_style=Wide Row  use_help_units=off  help='ADC voltage threshold above which ECU is considered powered'  units='ADC_counts'  use_header_enum=off  row_header_enum={}  col_header_enum={}  use_min_max=on  min_val=0  max_val=1023  use_precision=off  precision=''  gain=1  offset=0  exp=1  use_mototune_group=on  mototune_group=motohawk_vardec_config_group(group)
  motohawk_calibration1 : MotoHawk_lib/Calibration & Probing Blocks/motohawk_calibration  nam='Shutdown_Delay'  val=10  storage=Calibration  show_more=on  name_source=Use Parameter  data_type=Inherit via back propagation  read_level=1  write_level=1  ovr_cals=on  view_as=Number  enum_struct={'Disabled', 'Enabled'}  vector_style=Wide Row  use_help_units=on  help='ECU calibrateable shutdown delay'  units='Seconds'  use_header_enum=off  row_header_enum={}  col_header_enum={}  use_min_max=on  min_val=0  max_val=inf  use_precision=off  precision=''  gain=1  offset=0  exp=1  use_mototune_group=on  mototune_group=motohawk_vardec_config_group(group)
  motohawk_data_def : MotoHawk_lib/Data Storage Blocks/motohawk_data_def  nam='MPRD'  container_nam=''  data=false  typ=Inherit from 'Initial Value'  struct_nam='MyStruct'  storage=Volatile  outputRef=off  use_vardec=off  window=Display  read_level=1  write_level=(Read Only)  ovr_cals=on  view_as=Enumeration  enum_struct={'Disabled', 'Enabled'}  vector_style=Wide Row  use_help_units=on  help='Indicates whether the main power relay is active'  units=''  use_header_enum=off  row_header_enum={}  col_header_enum={}  use_min_max=off  min_val=-inf  max_val=inf  use_precision=off  precision=''  gain=1  offset=0  exp=1  use_mototune_group=on  mototune_group=group  eval_name=MPRD  data_stores=motohawk_sfun_data_def_data_stores  struct_instances=motohawk_sfun_data_def_struct_instances  vardecs=motohawk_sfun_data_def_vardecs
  motohawk_data_def1 : MotoHawk_lib/Data Storage Blocks/motohawk_data_def  nam='ShutDownTasksComplete'  container_nam=''  data=false  typ=boolean  struct_nam='MyStruct'  storage=Volatile  outputRef=off  use_vardec=off  window=Display  read_level=1  write_level=1  ovr_cals=on  view_as=Enumeration  enum_struct={'False', 'True'}  vector_style=Wide Row  use_help_units=off  help=''  units=''  use_header_enum=off  row_header_enum={}  col_header_enum={}  use_min_max=off  min_val=-inf  max_val=inf  use_precision=off  precision=''  gain=1  offset=0  exp=1  use_mototune_group=on  mototune_group='System | Main Power Relay'  eval_name=ShutDownTasksComplete  data_stores=motohawk_sfun_data_def_data_stores  struct_instances=motohawk_sfun_data_def_struct_instances  vardecs=motohawk_sfun_data_def_vardecs
  motohawk_data_read : MotoHawk_lib/Data Storage Blocks/motohawk_data_read  source=Lookup By Name  structure=Scalar  operation=Read entire data structure at once  sz_vec=4  sz_row=2  sz_col=3  typ=boolean  nam='ShutDownTasksComplete'  checkNull=on  struct_inst_name='Struct1'  struct_nam='MyStruct'
  motohawk_data_write : MotoHawk_lib/Data Storage Blocks/motohawk_data_write  source=Lookup By Name  structure=Scalar  operation=Write entire data structure at once  sz_vec=-1  sz_row=3  sz_col=2  typ=boolean  nam='MPRD'  checkNull=off  write_read_only=off  struct_inst_name='Struct1'  struct_name='MyStruct'
  motohawk_dout : MotoHawk_lib/Digital I//O Blocks/motohawk_dout  resource_name=[]  text_resource=MPRD  target=ECU565-128  use_diag=off  use_vardec=off  nam='DOUT'  read_level=1  write_level=1  group='System | I/O Pins | Outputs Config'
  motohawk_probe : MotoHawk_lib/Calibration & Probing Blocks/motohawk_probe  nam='ECUP_Enabled'  show_more=on  name_source=Use Parameter  read_level=1  view_as=Enumeration  enum_struct={'Disabled', 'Enabled'}  vector_style=Wide Row  use_help_units=off  help=''  units=''  use_header_enum=off  row_header_enum={}  col_header_enum={}  use_precision=off  precision=''  gain=1  offset=0  exp=1  use_mototune_group=on  mototune_group=group
  motohawk_restore_nvmem : MotoHawk_lib/Data Storage Blocks/motohawk_restore_nvmem  SystemSampleTime=-1
  motohawk_store_nvmem : MotoHawk_lib/Data Storage Blocks/motohawk_store_nvmem  SystemSampleTime=-1
  wires:
  Logical Operator/1 -> ShutDown Processes/2(Input State)
  ShutDown Processes/1(MPRD State) -> motohawk_data_write/1, motohawk_dout/1
  Relational Operator/1 -> Forced Shutdown Process/1(ECUP State), motohawk_probe/1, ECUP Latch/1(ECUP), Logical Operator3/1
  ECUP Latch/1(MPRDState) -> On Off Delay/1(In)
  Unit Delay5/1 -> ShutDown Processes/1(Manual Reset)
  Unit Delay4/1 -> Unit Delay5/1
  Unit Delay3/1 -> Unit Delay4/1
  Display Variable Event Function-Call1/1 -> motohawk_store_nvmem/Trigger
  Display Variable Event Function-Call/1 -> motohawk_restore_nvmem/Trigger
  Logical Operator1/1 -> Logical Operator/1
  On Off Delay/1(Out) -> Logical Operator/2
  Display Variable Event Boolean/1 -> Unit Delay3/1, Logical Operator1/1
  motohawk_calibration/1 -> Relational Operator/2
  motohawk_ain5/1 -> Relational Operator/1
  Logical Operator2/1 -> ECUP Latch/2(ShutDownTasks)
  Time Since Enabled (With Input)1/1 -> Relational Operator1/1
  motohawk_calibration1/1 -> Relational Operator1/2
  Relational Operator1/1 -> Logical Operator2/1
  Logical Operator3/1 -> Time Since Enabled (With Input)1/1, Logical Operator2/2
  motohawk_data_read/1 -> Logical Operator2/3
